simulink model "QuarterCar"  (R2023b)
settings: Solver=VariableStepAuto  StartTime=0.0  StopTime=10  RelTol=1e-3
settings Model: Creator=binyh  LastModifiedBy=binyh

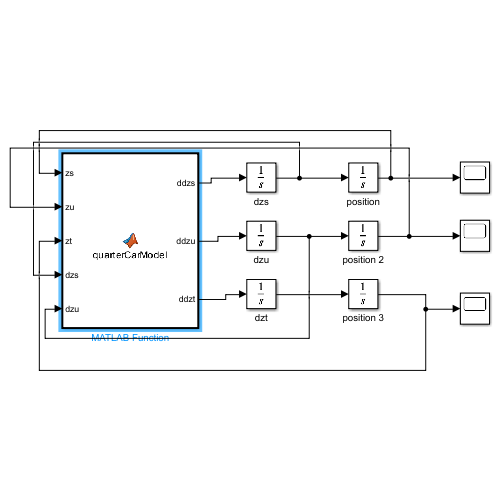
[thumbnail: Simulink's stored preview of the top-level diagram]
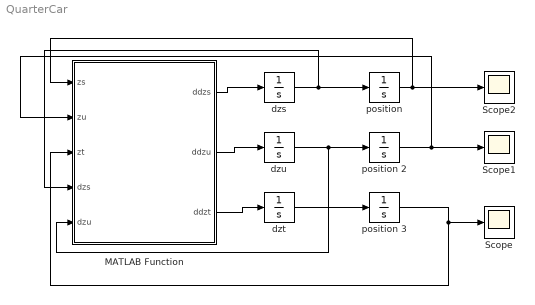
== system QuarterCar ==
  MATLAB Function : MATLAB Function  TreatAsAtomicUnit=on
  Scope : Scope
  Scope1 : Scope
  Scope2 : Scope
  dzs : Integrator
  dzt : Integrator
  dzu : Integrator
  position : Integrator  InitialCondition=1
  position 2 : Integrator  InitialCondition=0.5
  position 3 : Integrator
  wires:
  MATLAB Function/1(ddzs) -> dzs/1
  MATLAB Function/2(ddzu) -> dzu/1
  MATLAB Function/3(ddzt) -> dzt/1
  dzs/1 -> MATLAB Function/4(dzs), position/1
  dzu/1 -> MATLAB Function/5(dzu), position 2/1
  dzt/1 -> position 3/1
  position/1 -> Scope2/1, MATLAB Function/1(zs)
  position 2/1 -> Scope1/1, MATLAB Function/2(zu)
  position 3/1 -> Scope/1, MATLAB Function/3(zt)

== matlab function QuarterCar/MATLAB Function ==
  data: zs input; ddzs output; zu input; zt input; ddzu output; ddzt output; dzs input; dzu input
function [ddzs, ddzu, ddzt] = quarterCarModel(zs, zu, zt, dzs, dzu)
%basics - calculating the accelerations of sprung mass, unsprung mass, and
%tire of 1/4 of a car. 

    % parameters (arbitrary values)
    ms = 50; % sprung mass in kg (mass of the car body)
    mu = 10;  % unsprung mass in kg (mass of the wheel assembly)
    mt = 4;  % tire mass in kg
    ks = 50000; % spring constant of suspension in N/m
    kt = 127000; % spring constant of tire in N/m
    d = 0.5;   % damping coefficient in Ns/m

    % damping force = damping coefficient * velocity 

    ddzs = (ks * ((zu - zs)+0.5) - d * (dzu - dzs)) / ms;
    ddzu = (ks * ((zs - zu)-0.5) + (kt * ((zt - zu)+0.5)) - d * (dzs - dzu)) / mu;
    ddzt = kt * ((zu - zt)-0.5) / mt;

end

%   ddzs = (ks * ((zu - zs)+0.5) - d * (dzu - dzs)) / ms;
    %ddzu = (ks * ((zu - zs)+0.5) + kt * ((zt - zu)+0.5) - d * (dzu - dzs)) / mu;
    %ddzt = (kt * ((zu - zt)+0.5)) / mt;
